simulink model "serialComm_simulink"  (R2019a)
settings: Solver=FixedStepAuto  StartTime=0.0  StopTime=10.0  FixedStep=1E-3  RelTol=1e-3  EnableMultiTasking=on
libraries: frdmk64flib x2
settings Model: ExtModeTrigDuration=5  Creator=Laura  LastModifiedBy=Laura
settings OptimizationCC: EnhancedBackFolding=on  PassReuseOutputArgsAs=Individual arguments  MaxStackSize=64  OptimizeBlockOrder=speed  DifferentSizesBufferReuse=on  OptimizationCustomize=off
settings DebuggingCC: ParameterTunabilityLossMsg=error
settings HardwareCC: ProdBitPerPointer=32  ProdBitPerSizeT=32  ProdBitPerPtrDiffT=32  ProdLargestAtomicInteger=Long  ProdLargestAtomicFloat=Double  ProdWordSize=32  ProdHWDeviceType=ARM Compatible->ARM Cortex
settings SFSimCC: MATLABDynamicMemAlloc=off
settings RTWCC: SystemTargetFile=ert.tlc  HardwareBoard=NXP FRDM-K64F  TLCOptions="-aInlineSetEventsForThisBaseRateFcn=TLC_FALSE -aSuppressMultiTaskScheduler=TLC_FALSE  -aRateBasedStepFcn=0"  TemplateMakefile=ert_default_tmf  GenerateReport=on  Toolchain=GNU Tools for ARM Embedded Processors  IncludeHyperlinkInReport=on  LaunchReport=on  GenerateTraceInfo=on  GenerateTraceReport=on  GenerateTraceReportSl=on  GenerateTraceReportSf=on  GenerateTraceReportEml=on
settings CodeAppCC: ForceParamTrailComments=on  IgnoreCustomStorageClasses=off  OperatorAnnotations=on  SimulinkDataObjDesc=on  SFDataObjDesc=on  InsertBlockDesc=on

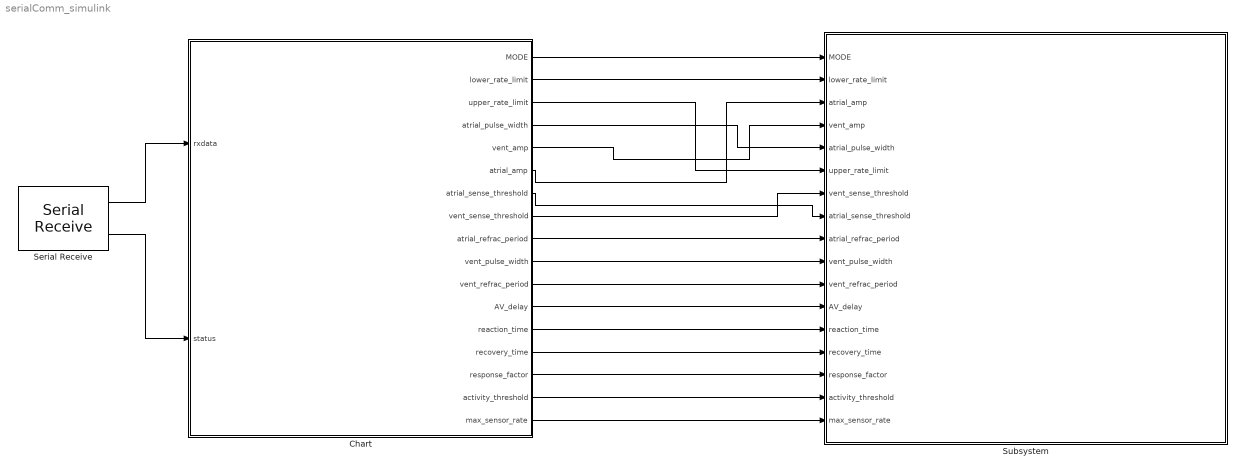
== system serialComm_simulink ==
  Chart : Stateflow chart  BlockKeywords=__PRM__SERIALIZED__DATA__:Stateflow Chart,Stateflow Diagram  TreatAsAtomicUnit=on
  Serial Receive : frdmk64flib/Serial Receive  SCIModule=0  Baudrate=uint32(9600)  Parity=None  StopBits=1  HardwareFlowControl=None  ByteOrder=LittleEndian  DataType=uint8  DataLength=55  BlockingMode=off  OutputStatus=on  SampleTime=-1
      settings: SourceProductName=Simulink Coder Support Package for NXP FRDM-K64F Board
  Subsystem : Subsystem
  wires:
  Serial Receive/1 -> Chart/1(rxdata)
  Serial Receive/2 -> Chart/2(status)
  Chart/2(lower_rate_limit) -> Subsystem/2(lower_rate_limit)
  Chart/6(atrial_amp) -> Subsystem/3(atrial_amp)
  Chart/5(vent_amp) -> Subsystem/4(vent_amp)
  Chart/4(atrial_pulse_width) -> Subsystem/5(atrial_pulse_width)
  Chart/3(upper_rate_limit) -> Subsystem/6(upper_rate_limit)
  Chart/7(atrial_sense_threshold) -> Subsystem/8(atrial_sense_threshold)
  Chart/8(vent_sense_threshold) -> Subsystem/7(vent_sense_threshold)
  Chart/9(atrial_refrac_period) -> Subsystem/9(atrial_refrac_period)
  Chart/10(vent_pulse_width) -> Subsystem/10(vent_pulse_width)
  Chart/11(vent_refrac_period) -> Subsystem/11(vent_refrac_period)
  Chart/12(AV_delay) -> Subsystem/12(AV_delay)
  Chart/13(reaction_time) -> Subsystem/13(reaction_time)
  Chart/14(recovery_time) -> Subsystem/14(recovery_time)
  Chart/15(response_factor) -> Subsystem/15(response_factor)
  Chart/16(activity_threshold) -> Subsystem/16(activity_threshold)
  Chart/17(max_sensor_rate) -> Subsystem/17(max_sensor_rate)
  Chart/1(MODE) -> Subsystem/1(MODE)

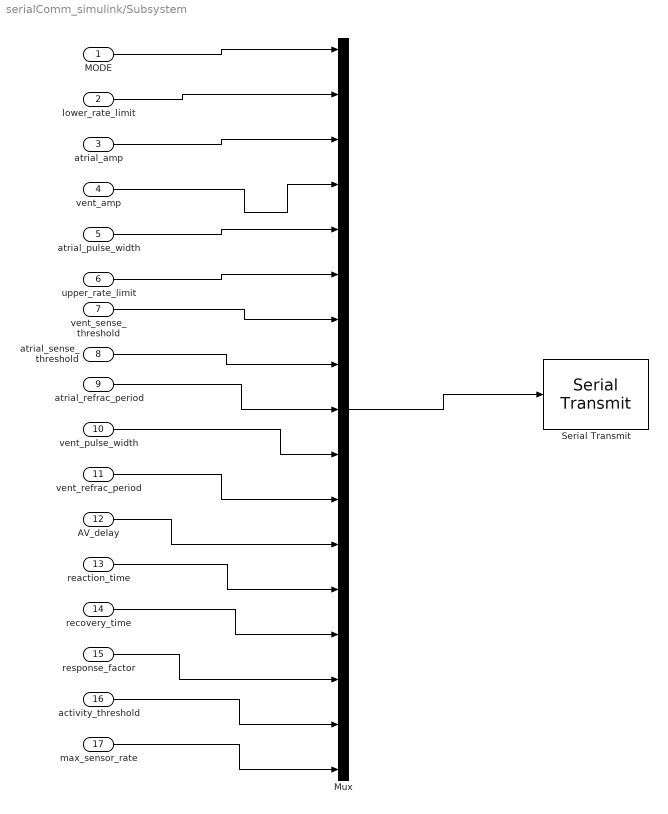
== system serialComm_simulink/Subsystem ==
  MODE : Inport
  lower_rate_limit : Inport  Port=2
  atrial_amp : Inport  Port=3
  vent_amp : Inport  Port=4
  atrial_pulse_width : Inport  Port=5
  upper_rate_limit : Inport  Port=6
  vent_sense_threshold : Inport  Port=7
  atrial_sense_threshold : Inport  Port=8
  atrial_refrac_period : Inport  Port=9
  vent_pulse_width : Inport  Port=10
  vent_refrac_period : Inport  Port=11
  AV_delay : Inport  Port=12
  reaction_time : Inport  Port=13
  recovery_time : Inport  Port=14
  response_factor : Inport  Port=15
  activity_threshold : Inport  Port=16
  max_sensor_rate : Inport  Port=17
  Mux : Mux  Inputs=17
  Serial Transmit : frdmk64flib/Serial Transmit  SCIModule=0  Baudrate=uint32(9600)  Parity=None  StopBits=1  HardwareFlowControl=None  ByteOrder=LittleEndian  BlockingMode=on  OutputStatus=off
      settings: SourceProductName=Simulink Coder Support Package for NXP FRDM-K64F Board
  wires:
  Mux/1 -> Serial Transmit/1
  MODE/1 -> Mux/1
  lower_rate_limit/1 -> Mux/2
  atrial_amp/1 -> Mux/3
  vent_amp/1 -> Mux/4
  atrial_pulse_width/1 -> Mux/5
  upper_rate_limit/1 -> Mux/6
  vent_sense_threshold/1 -> Mux/7
  atrial_sense_threshold/1 -> Mux/8
  atrial_refrac_period/1 -> Mux/9
  vent_pulse_width/1 -> Mux/10
  vent_refrac_period/1 -> Mux/11
  AV_delay/1 -> Mux/12
  reaction_time/1 -> Mux/13
  recovery_time/1 -> Mux/14
  response_factor/1 -> Mux/15
  activity_threshold/1 -> Mux/16
  max_sensor_rate/1 -> Mux/17

== stateflow chart serialComm_simulink/Chart ==
  state SET_PARAMS
    %we assume this is the order that the data is sent in
    entry:
    MODE = rxdata(1)
    lower_rate_limit = typecast(rxdata(2:3), 'uint16')
    upper_rate_limit = typecast(rxdata(4:5), 'uint16')
    atrial_amp = typecast(rxdata(6:13), 'double')
    vent_amp = typecast(rxdata(14:21), 'double')
    atrial_pulse_width = typecast(rxdata(22:23), 'uint16')
    vent_pulse_width = typecast(rxdata(24:25), 'uint16')
    atrial_sense_threshold = typecast(rxdata(26:33), 'double')
    vent_sense_threshold = typecast(rxdata(34:41), 'double')
    atrial_refrac_period = typecast(rxdata(42:43), 'uint16')
    vent_refrac_period = typecast(rxdata(44:45), 'uint16')
    AV_delay = typecast(rxdata(46:47), 'uint16')
    reaction_time = typecast(rxdata(48:49), 'uint16')
    recovery_time = typecast(rxdatta(50:51), 'uint16')
    response_factor = rxdata(52)
    activity_threshold = rxdata(53)
    max_sensor_rate = typecast(rxdata(54:55), 'uint16')
  state INITIAL
    entry:
    MODE = 0
    lower_rate_limit = 60
    upper_rate_limit = 150
    atrial_amp = 3.3
    vent_amp = 3.3
    atrial_pulse_width = 10
    vent_pulse_width = 10
    atrial_sense_threshold = 2.75
    vent_sense_threshold = 2.75
    atrial_refrac_period = 100
    vent_refrac_period = 100
    AV_delay = 1
    reaction_time = 0 %unknown
    recovery_time = 0 %unknown
    response_factor = 0 %unknown
    activity_threshold = 0 %unknown
    max_sensor_rate = 0 %unknown
  state STANDBY
    %Waiting for COM
  state SEND_PARAMS
    entry:
  (default) -> INITIAL
  (junction 8) -> STANDBY [order 2] : [status == 0]
  STANDBY -> (junction 8)
  (junction 8) -> SET_PARAMS [order 1] : [status == 1]
  INITIAL -> STANDBY
  data: rxdata input; status input; MODE output; lower_rate_limit output; upper_rate_limit output; atrial_pulse_width output; vent_amp output; atrial_amp output; atrial_sense_threshold output; vent_sense_threshold output; atrial_refrac_period output; vent_pulse_width output; vent_refrac_period output; AV_delay output; reaction_time output; recovery_time output; response_factor output; activity_threshold output; max_sensor_rate output
